simulink model "tank_level_control"  (R2025a)
settings: Solver=ode45  StartTime=0.0  StopTime=600  RelTol=1e-3
libraries: slpidlib x1
settings Model: Creator=gigass  LastModifiedBy=gigass

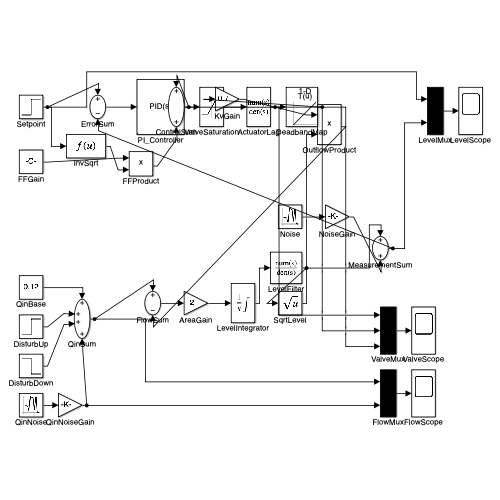
[thumbnail: Simulink's stored preview of the top-level diagram]
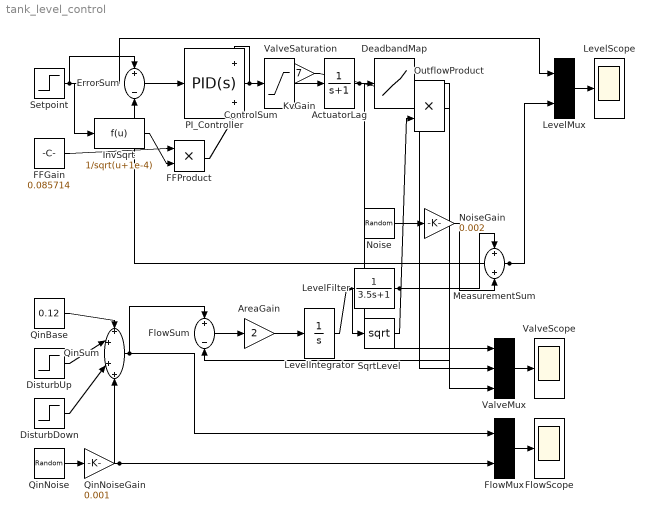
== system tank_level_control ==
  ActuatorLag : TransferFcn  Denominator=[1 1]
  AreaGain : Gain  Gain=2
  ControlSum : Sum
  DeadbandMap : Lookup_n-D  NumberOfTableDimensions=1  BreakpointsForDimension1=[0 1]  Table=[0 1]  InternalRulePriority=Speed  RndMeth=Simplest
  DisturbDown : Step  Time=450  After=-0.04  SampleTime=0
  DisturbUp : Step  Time=350  After=0.04  SampleTime=0
  ErrorSum : Sum  Inputs=+-
  FFGain : Constant  Value=0.085714
  FFProduct : Product  Inputs=**
  FlowMux : Mux  Inputs=2
  FlowScope : Scope
  FlowSum : Sum  Inputs=+-
  InvSqrt : Fcn  Expr=1/sqrt(u+1e-4)
  KvGain : Gain  Gain=0.7
  LevelFilter : TransferFcn  Denominator=[3.5 1]
  LevelIntegrator : Integrator  InitialCondition=0.5  LimitOutput=on  UpperSaturationLimit=2  LowerSaturationLimit=0
  LevelMux : Mux  Inputs=2
  LevelScope : Scope
  MeasurementSum : Sum
  Noise : RandomNumber  SampleTime=0.01
  NoiseGain : Gain  Gain=0.002
  OutflowProduct : Product  Inputs=**
  PI_Controller : slpidlib/PID Controller  Controller=PID  Form=Parallel  TimeDomain=Continuous-time  UseExternalTs=off  SampleTime=-1  IntegratorMethod=Forward Euler  FilterMethod=Forward Euler  ControllerParametersSource=internal  P=1.8  I=0.12  UseKiTs=off  D=0  UseExternalDerivativeSource=off  N=100  UseFilter=on  TunerSelectOption=Transfer Function Based (PID Tuner App)  InitialConditionSource=internal  InitialConditionForIntegrator=0  InitialConditionForFilter=0  DifferentiatorICPrevScaledInput=0  ExternalReset=none  TrackingMode=off  Kt=1  LimitOutput=off  SatLimitsSource=internal  UpperSaturationLimit=inf  LowerSaturationLimit=-inf  LinearizeAsGain=on  AntiWindupMode=none  Kb=1  LimitIntegrator=off  UpperIntegratorSaturationLimit=inf  LowerIntegratorSaturationLimit=-inf  POutMin=[]  POutMax=[]  IOutMin=[]  IOutMax=[]  DOutMin=[]  DOutMax=[]  NOutMin=[]  NOutMax=[]  SumOutMin=[]  SumOutMax=[]  SaturationOutMin=[]  SaturationOutMax=[]  PParamMin=[]  PParamMax=[]  IParamMin=[]  IParamMax=[]  DParamMin=[]  DParamMax=[]  NParamMin=[]  NParamMax=[]  KbParamMin=[]  KbParamMax=[]  KtParamMin=[]  KtParamMax=[]  KbOutMin=[]  KbOutMax=[]  KtOutMin=[]  KtOutMax=[]  IntegratorOutMin=[]  IntegratorOutMax=[]  FilterOutMin=[]  FilterOutMax=[]  SumI1OutMin=[]  SumI1OutMax=[]  SumI2OutMin=[]  SumI2OutMax=[]  SumI3OutMin=[]  SumI3OutMax=[]  SumI4OutMin=[]  SumI4OutMax=[]  SumDOutMin=[]  SumDOutMax=[]  DifferentiatorOutMin=[]  DifferentiatorOutMax=[]  FilterDiffOutCoefMin=[]  FilterDiffOutCoefMax=[]  ReciprocalOutMin=[]  ReciprocalOutMax=[]  SumDenOutMin=[]  SumDenOutMax=[]  SumNumOutMin=[]  SumNumOutMax=[]  DivideOutMin=[]  DivideOutMax=[]  UdiffTsProdOutMin=[]  UdiffTsProdOutMax=[]  NTsProdOutMin=[]  NTsProdOutMax=[]  UintegralTsProdOutMin=[]  UintegralTsProdOutMax=[]  UngainTsProdOutMin=[]  UngainTsProdOutMax=[]  ClampingZeroOutDataTypeStr=Inherit: Inherit via back propagation  ClampingZeroOutMin=[]  ClampingZeroOutMax=[]  FilterDenConstantOutDataTypeStr=Inherit: Inherit via back propagation  FilterDenConstantOutMin=[]  FilterDenConstantOutMax=[]  PCopyOutDataTypeStr=Inherit: Inherit via back propagation  PCopyOutMin=[]  PCopyOutMax=[]  NCopyOutDataTypeStr=Inherit: Inherit via back propagation  NCopyOutMin=[]  NCopyOutMax=[]  IntegratorContinuousStateAttributes=''  IntegratorStateMustResolveToSignalObject=off  IntegratorRTWStateStorageClass=Auto  FilterContinuousStateAttributes=''  FilterStateMustResolveToSignalObject=off  FilterRTWStateStorageClass=Auto  ParallelPVariant=InternalParameters  IdealPVariant=Disabled  IVariant=InternalParameters  DVariant=InternalParameters  IntegratorVariant=Continuous  SatVariant=Disabled  AWVariant=Passthrough  PCopyVariant=Disabled  TRVariant=Disabled  FdbkBlocksVariant=Forward  IdealPFdbkVariant=Disabled  SatFdbkVariant=Disabled  DerivativeFilterVariant=ContFilter  NVariant=InternalParameters  NCopyVariant=Disabled  FilterICVariant=InternalICsFilter  IntegratorICVariant=InternalICs  ExternalResetVariant=Disabled  TRSumVariant=Passthrough  SumFdbkVariant=Disabled  SumVariant=Sum_PID  TsampFilterVariant=InternalTs  TsampNgainVariant=Passthrough  TsampIntegralVariant=Disabled_SignalSpec  ExternalSaturationOutDataTypeStr=Inherit: Same as second input  DerivativeSourceVariant=ErrorSignal  PreIntVariant=InternalPreInt
  QinBase : Constant  Value=0.12
  QinNoise : RandomNumber  Seed=1  SampleTime=0.1
  QinNoiseGain : Gain  Gain=0.001
  QinSum : Sum  Inputs=++++
  Setpoint : Step  Time=200  Before=0.5  After=0.65  SampleTime=0
  SqrtLevel : Math  Operator=sqrt
  ValveMux : Mux  Inputs=3
  ValveSaturation : Saturate  UpperLimit=1  LowerLimit=0
  ValveScope : Scope
  wires:
  Setpoint/1 -> ErrorSum/1, InvSqrt/1, LevelMux/1
  FFGain/1 -> FFProduct/1
  InvSqrt/1 -> FFProduct/2
  FFProduct/1 -> ControlSum/2
  MeasurementSum/1 -> ErrorSum/2, LevelMux/2
  ErrorSum/1 -> PI_Controller/1
  PI_Controller/1 -> ControlSum/1
  ControlSum/1 -> ValveSaturation/1, ValveMux/1
  ValveSaturation/1 -> ActuatorLag/1
  ActuatorLag/1 -> DeadbandMap/1, ValveMux/2
  DeadbandMap/1 -> KvGain/1, ValveMux/3
  KvGain/1 -> OutflowProduct/1
  SqrtLevel/1 -> OutflowProduct/2
  OutflowProduct/1 -> FlowSum/2
  QinBase/1 -> QinSum/1
  DisturbUp/1 -> QinSum/2
  DisturbDown/1 -> QinSum/3
  QinNoise/1 -> QinNoiseGain/1
  QinNoiseGain/1 -> QinSum/4, FlowMux/2
  QinSum/1 -> FlowSum/1, FlowMux/1
  FlowSum/1 -> AreaGain/1
  AreaGain/1 -> LevelIntegrator/1
  LevelIntegrator/1 -> LevelFilter/1
  LevelFilter/1 -> SqrtLevel/1, MeasurementSum/1
  Noise/1 -> NoiseGain/1
  NoiseGain/1 -> MeasurementSum/2
  LevelMux/1 -> LevelScope/1
  ValveMux/1 -> ValveScope/1
  FlowMux/1 -> FlowScope/1
